simulink model "Appl_HeatAdj_CtrlModel"  (R2018b)
settings: configuration reference "CodeConfig_10_ms" (kept outside this file)
undefined symbols (not defined in the file): CAL_LEVEL3_TIMEOUT, CAL_SW_20min_TIMEOUT, D_1stLevel_36, D_2ndLevel_39, D_3rdLevel_45, D_3rdLevel_48, D_DRVHEAT_PID_D, D_DRVHEAT_PID_I, D_DRVHEAT_PID_P, D_HEAT_HEAT_DEF, D_SwsLevel_Temp, FALSE, TRUE
libraries: DareLib x111, simulink x1
(part 3 of 6)

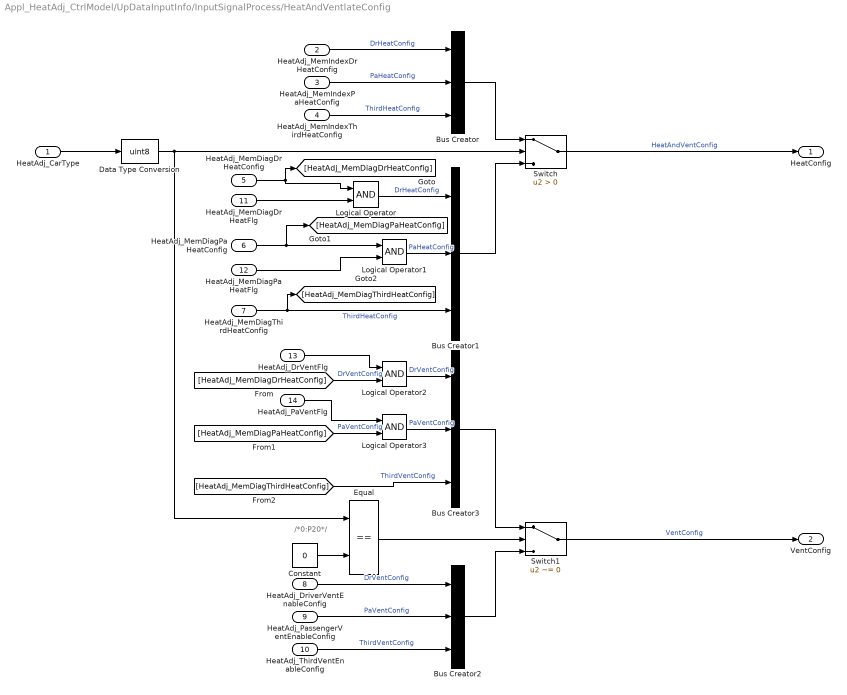
== system Appl_HeatAdj_CtrlModel/UpDataInputInfo/InputSignalProcess/HeatAndVentlateConfig ==
  note: /*0:P20*/
  HeatAdj_CarType : Inport
  HeatAdj_MemIndexDrHeatConfig : Inport  Port=2
  HeatAdj_MemIndexPaHeatConfig : Inport  Port=3
  HeatAdj_MemIndexThirdHeatConfig : Inport  Port=4
  HeatAdj_MemDiagDrHeatConfig : Inport  Port=5
  HeatAdj_MemDiagPaHeatConfig : Inport  Port=6
  HeatAdj_MemDiagThirdHeatConfig : Inport  Port=7
  HeatAdj_DriverVentEnableConfig : Inport  Port=8
  HeatAdj_PassengerVentEnableConfig : Inport  Port=9
  HeatAdj_ThirdVentEnableConfig : Inport  Port=10
  HeatAdj_MemDiagDrHeatFlg : Inport  Port=11
  HeatAdj_MemDiagPaHeatFlg : Inport  Port=12
  HeatAdj_DrVentFlg : Inport  Port=13
  HeatAdj_PaVentFlg : Inport  Port=14
  Bus Creator{,1..3} (4 alike) : BusCreator  Inputs=3
  Constant : Constant  Value=0  OutDataTypeStr=uint8
  Data Type Conversion : DataTypeConversion  OutDataTypeStr=uint8
  Equal : RelationalOperator  Operator===  OutDataTypeStr=boolean  RndMeth=Simplest
  Logical Operator{,1..3} (4 alike) : Logic  AllPortsSameDT=off  OutDataTypeStr=boolean
  Switch : Switch  Criteria=u2 > Threshold  OutDataTypeStr=uint8
  Switch1 : Switch  Criteria=u2 ~= 0
  HeatConfig : Outport
  VentConfig : Outport  Port=2
  wires:
  HeatAdj_CarType/1 -> Data Type Conversion/1
  HeatAdj_MemIndexDrHeatConfig/1 -> Bus Creator/1  "DrHeatConfig"
  HeatAdj_MemIndexPaHeatConfig/1 -> Bus Creator/2  "PaHeatConfig"
  HeatAdj_MemIndexThirdHeatConfig/1 -> Bus Creator/3  "ThirdHeatConfig"
  Bus Creator/1 -> Switch/1
  Bus Creator1/1 -> Switch/3
  HeatAdj_MemDiagDrHeatConfig/1 -> Logical Operator/1, [HeatAdj_MemDiagDrHeatConfig]
  HeatAdj_MemDiagPaHeatConfig/1 -> Logical Operator1/1, [HeatAdj_MemDiagPaHeatConfig]
  HeatAdj_MemDiagThirdHeatConfig/1 -> [HeatAdj_MemDiagThirdHeatConfig], Bus Creator1/3  "ThirdHeatConfig"
  Constant/1 -> Equal/2
  Equal/1 -> Switch1/2
  HeatAdj_DriverVentEnableConfig/1 -> Bus Creator2/1  "DrVentConfig"
  HeatAdj_PassengerVentEnableConfig/1 -> Bus Creator2/2  "PaVentConfig"
  HeatAdj_ThirdVentEnableConfig/1 -> Bus Creator2/3  "ThirdVentConfig"
  Bus Creator2/1 -> Switch1/3
  Switch/1 -> HeatConfig/1  "HeatAndVentConfig"
  Data Type Conversion/1 -> Switch/2, Equal/1
  Switch1/1 -> VentConfig/1  "VentConfig"
  [HeatAdj_MemDiagThirdHeatConfig] -> Bus Creator3/3  "ThirdVentConfig"
  [HeatAdj_MemDiagPaHeatConfig] -> Logical Operator3/2  "PaVentConfig"
  [HeatAdj_MemDiagDrHeatConfig] -> Logical Operator2/2  "DrVentConfig"
  Bus Creator3/1 -> Switch1/1
  HeatAdj_MemDiagDrHeatFlg/1 -> Logical Operator/2
  Logical Operator/1 -> Bus Creator1/1  "DrHeatConfig"
  HeatAdj_MemDiagPaHeatFlg/1 -> Logical Operator1/2
  Logical Operator1/1 -> Bus Creator1/2  "PaHeatConfig"
  HeatAdj_DrVentFlg/1 -> Logical Operator2/1
  Logical Operator2/1 -> Bus Creator3/1  "DrVentConfig"
  Logical Operator3/1 -> Bus Creator3/2  "PaVentConfig"
  HeatAdj_PaVentFlg/1 -> Logical Operator3/1

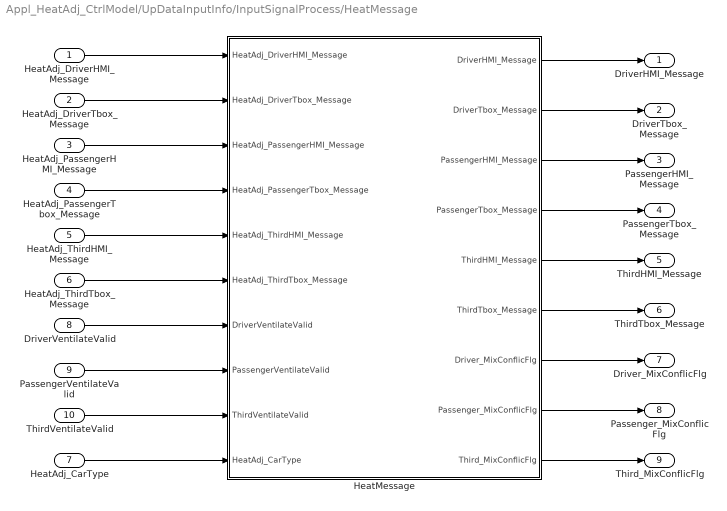
== system Appl_HeatAdj_CtrlModel/UpDataInputInfo/InputSignalProcess/HeatMessage ==
  HeatAdj_DriverHMI_Message : Inport
  HeatAdj_DriverTbox_Message : Inport  Port=2
  HeatAdj_PassengerHMI_Message : Inport  Port=3
  HeatAdj_PassengerTbox_Message : Inport  Port=4
  HeatAdj_ThirdHMI_Message : Inport  Port=5
  HeatAdj_ThirdTbox_Message : Inport  Port=6
  HeatAdj_CarType : Inport  Port=7
  DriverVentilateValid : Inport  Port=8
  PassengerVentilateValid : Inport  Port=9
  ThirdVentilateValid : Inport  Port=10
  HeatMessage : Stateflow chart  TreatAsAtomicUnit=on
  DriverHMI_Message : Outport
  DriverTbox_Message : Outport  Port=2
  PassengerHMI_Message : Outport  Port=3
  PassengerTbox_Message : Outport  Port=4
  ThirdHMI_Message : Outport  Port=5
  ThirdTbox_Message : Outport  Port=6
  Driver_MixConflicFlg : Outport  Port=7
  Passenger_MixConflicFlg : Outport  Port=8
  Third_MixConflicFlg : Outport  Port=9
  wires:
  HeatMessage/4(PassengerTbox_Message) -> PassengerTbox_Message/1
  HeatMessage/5(ThirdHMI_Message) -> ThirdHMI_Message/1
  HeatMessage/6(ThirdTbox_Message) -> ThirdTbox_Message/1
  ThirdVentilateValid/1 -> HeatMessage/9(ThirdVentilateValid)
  HeatAdj_DriverTbox_Message/1 -> HeatMessage/2(HeatAdj_DriverTbox_Message)
  HeatAdj_DriverHMI_Message/1 -> HeatMessage/1(HeatAdj_DriverHMI_Message)
  HeatAdj_PassengerHMI_Message/1 -> HeatMessage/3(HeatAdj_PassengerHMI_Message)
  HeatAdj_PassengerTbox_Message/1 -> HeatMessage/4(HeatAdj_PassengerTbox_Message)
  HeatAdj_ThirdHMI_Message/1 -> HeatMessage/5(HeatAdj_ThirdHMI_Message)
  PassengerVentilateValid/1 -> HeatMessage/8(PassengerVentilateValid)
  HeatAdj_ThirdTbox_Message/1 -> HeatMessage/6(HeatAdj_ThirdTbox_Message)
  DriverVentilateValid/1 -> HeatMessage/7(DriverVentilateValid)
  HeatMessage/1(DriverHMI_Message) -> DriverHMI_Message/1
  HeatMessage/2(DriverTbox_Message) -> DriverTbox_Message/1
  HeatMessage/3(PassengerHMI_Message) -> PassengerHMI_Message/1
  HeatAdj_CarType/1 -> HeatMessage/10(HeatAdj_CarType)
  HeatMessage/7(Driver_MixConflicFlg) -> Driver_MixConflicFlg/1
  HeatMessage/8(Passenger_MixConflicFlg) -> Passenger_MixConflicFlg/1
  HeatMessage/9(Third_MixConflicFlg) -> Third_MixConflicFlg/1

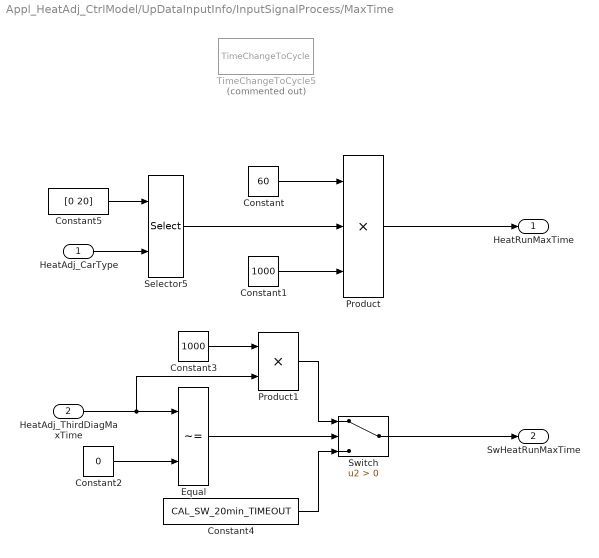
== system Appl_HeatAdj_CtrlModel/UpDataInputInfo/InputSignalProcess/MaxTime ==
  HeatAdj_CarType : Inport
  HeatAdj_ThirdDiagMaxTime : Inport  Port=2
  Constant : Constant  Value=60  OutDataTypeStr=uint32
  Constant1 : Constant  Value=1000  OutDataTypeStr=uint32
  Constant2 : Constant  Value=0  OutDataTypeStr=uint32
  Constant3 : Constant  Value=1000  OutDataTypeStr=uint32
  Constant4 : Constant  Value=CAL_SW_20min_TIMEOUT  OutDataTypeStr=uint32
  Constant5 : Constant  Value=[0 20]  OutDataTypeStr=uint32
  Equal : RelationalOperator  Operator=~=  OutDataTypeStr=boolean  RndMeth=Simplest
  Product : Product  Inputs=3  OutDataTypeStr=uint32
  Product1 : Product  OutDataTypeStr=uint32
  Selector5 : Selector  IndexMode=Zero-based  InputPortWidth=2  IndexOptions=Index vector (port)  Indices=[1 3]  OutputSizes=1
  Switch : Switch  Criteria=u2 > Threshold
  TimeChangeToCycle5 : DareLib/Dare/TimeChangeToCycle  Description=时间转成执行周期  Commented=on  Sec=60  Msec=1000  Cycle=CAL_HeatAdjCycle_10ms
      settings: AttributesFormatString=%<Description>  SourceProductName=Dare Library
  HeatRunMaxTime : Outport
  SwHeatRunMaxTime : Outport  Port=2
  wires:
  HeatAdj_CarType/1 -> Selector5/2
  Constant5/1 -> Selector5/1
  Selector5/1 -> Product/2
  Constant/1 -> Product/1
  Constant1/1 -> Product/3
  Product/1 -> HeatRunMaxTime/1
  HeatAdj_ThirdDiagMaxTime/1 -> Product1/2, Equal/1
  Constant2/1 -> Equal/2
  Equal/1 -> Switch/2
  Product1/1 -> Switch/1
  Constant3/1 -> Product1/1
  Constant4/1 -> Switch/3
  Switch/1 -> SwHeatRunMaxTime/1

== system Appl_HeatAdj_CtrlModel/UpDataInputInfo/InputSignalProcess/RemoteMode ==
  HeatAdj_RemoteEnableConfig : Inport
  HeatAdj_TboxRemoteSts : Inport  Port=2
  HeatAdj_RemoteMsgLostFlag : Inport  Port=3
  RemoteMode : Stateflow chart  TreatAsAtomicUnit=on
  RemoteModeFlag : Outport
  wires:
  HeatAdj_TboxRemoteSts/1 -> RemoteMode/2(HeatAdj_TboxRemoteSts)
  HeatAdj_RemoteEnableConfig/1 -> RemoteMode/1(HeatAdj_RemoteEnableConfig)
  HeatAdj_RemoteMsgLostFlag/1 -> RemoteMode/3(HeatAdj_RemoteMsgLostFlag)
  RemoteMode/1(RemoteModeFlag) -> RemoteModeFlag/1

== system Appl_HeatAdj_CtrlModel/UpDataInputInfo/InputSignalProcess/VehRunSta ==
  HeatAdj_PlatformVehicleEnableConfig : Inport
  HeatAdj_P20_PHEV_EngineCfg : Inport  Port=2
  HeatAdj_VCU_VehRunSta : Inport  Port=3
  HeatAdj_CarType : Inport  Port=4
  VehicleRunStatus : Stateflow chart  TreatAsAtomicUnit=on
  "VehicleRunFlag " : Outport
  wires:
  HeatAdj_VCU_VehRunSta/1 -> VehicleRunStatus/3(HeatAdj_VCU_VehRunSta)
  HeatAdj_PlatformVehicleEnableConfig/1 -> VehicleRunStatus/1(HeatAdj_PlatformVehicleEnableConfig)
  HeatAdj_P20_PHEV_EngineCfg/1 -> VehicleRunStatus/2(HeatAdj_P20_PHEV_EngineCfg)
  VehicleRunStatus/1(VehicleRunFlag) -> "VehicleRunFlag "/1
  HeatAdj_CarType/1 -> VehicleRunStatus/4(HeatAdj_CarType)

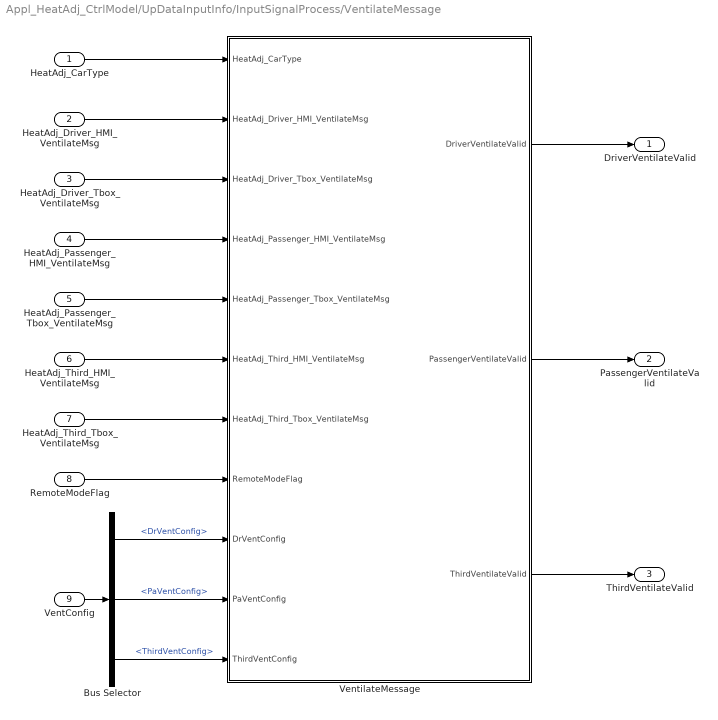
== system Appl_HeatAdj_CtrlModel/UpDataInputInfo/InputSignalProcess/VentilateMessage ==
  HeatAdj_CarType : Inport
  HeatAdj_Driver_HMI_VentilateMsg : Inport  Port=2
  HeatAdj_Driver_Tbox_VentilateMsg : Inport  Port=3
  HeatAdj_Passenger_HMI_VentilateMsg : Inport  Port=4
  HeatAdj_Passenger_Tbox_VentilateMsg : Inport  Port=5
  HeatAdj_Third_HMI_VentilateMsg : Inport  Port=6
  HeatAdj_Third_Tbox_VentilateMsg : Inport  Port=7
  RemoteModeFlag : Inport  Port=8
  VentConfig : Inport  Port=9
  Bus Selector : BusSelector  OutputSignals=DrVentConfig,PaVentConfig,ThirdVentConfig
  VentilateMessage : Stateflow chart  TreatAsAtomicUnit=on
  DriverVentilateValid : Outport
  PassengerVentilateValid : Outport  Port=2
  ThirdVentilateValid : Outport  Port=3
  wires:
  HeatAdj_Driver_HMI_VentilateMsg/1 -> VentilateMessage/2(HeatAdj_Driver_HMI_VentilateMsg)
  HeatAdj_CarType/1 -> VentilateMessage/1(HeatAdj_CarType)
  HeatAdj_Driver_Tbox_VentilateMsg/1 -> VentilateMessage/3(HeatAdj_Driver_Tbox_VentilateMsg)
  HeatAdj_Passenger_HMI_VentilateMsg/1 -> VentilateMessage/4(HeatAdj_Passenger_HMI_VentilateMsg)
  HeatAdj_Passenger_Tbox_VentilateMsg/1 -> VentilateMessage/5(HeatAdj_Passenger_Tbox_VentilateMsg)
  RemoteModeFlag/1 -> VentilateMessage/8(RemoteModeFlag)
  HeatAdj_Third_HMI_VentilateMsg/1 -> VentilateMessage/6(HeatAdj_Third_HMI_VentilateMsg)
  HeatAdj_Third_Tbox_VentilateMsg/1 -> VentilateMessage/7(HeatAdj_Third_Tbox_VentilateMsg)
  VentilateMessage/1(DriverVentilateValid) -> DriverVentilateValid/1
  VentilateMessage/2(PassengerVentilateValid) -> PassengerVentilateValid/1
  VentilateMessage/3(ThirdVentilateValid) -> ThirdVentilateValid/1
  VentConfig/1 -> Bus Selector/1
  Bus Selector/1 -> VentilateMessage/9(DrVentConfig)  "<DrVentConfig>"
  Bus Selector/2 -> VentilateMessage/10(PaVentConfig)  "<PaVentConfig>"
  Bus Selector/3 -> VentilateMessage/11(ThirdVentConfig)  "<ThirdVentConfig>"

== system Appl_HeatAdj_CtrlModel/LogicCtrl/LocalAdjustCtrl/LimitDeal/TimeoutFunction/Timeout/D_HAL_GET_CUR_MS_TS ==
  f : TriggerPort  TriggerType=function-call  VariantControl=(inherit)
      settings: CopyFcn=Stateflow.SLINSF.SimulinkMan.removeBlockPreDeleteFcn  PreDeleteFcn=Stateflow.SLINSF.SimulinkMan.unsafePredeleteFcn
  DrAdj_LenAdjSize : DareLib/Dare/getAPI_type  g_funcname=D_HAL_GET_CUR_MS_TS  g_param=""  g_type=uint32  g_size=-1
      settings: SourceProductName=Dare Library
  Ts : Outport
  wires:
  DrAdj_LenAdjSize/1 -> Ts/1  "D_HAL_GET_CUR_MS_TS"

== system Appl_HeatAdj_CtrlModel/LogicCtrl/LocalAdjustCtrl/LimitDeal/TimeoutFunction/Timeout/TimeDiffTs ==
  lastTs : Inport
  Ts : Inport  Port=2
  f : TriggerPort  TriggerType=function-call  VariantControl=(inherit)
      settings: CopyFcn=Stateflow.SLINSF.SimulinkMan.removeBlockPreDeleteFcn  PreDeleteFcn=Stateflow.SLINSF.SimulinkMan.unsafePredeleteFcn
  Chart : Stateflow chart  TreatAsAtomicUnit=on
  OutTs : Outport
  wires:
  lastTs/1 -> Chart/1(lastTs)
  Ts/1 -> Chart/2(Ts)
  Chart/1(OutTs) -> OutTs/1

== system Appl_HeatAdj_CtrlModel/LogicCtrl/LocalAdjustCtrl/LimitDeal/TimeoutFunction1/Timeout/D_HAL_GET_CUR_MS_TS ==
  f : TriggerPort  TriggerType=function-call  VariantControl=(inherit)
      settings: CopyFcn=Stateflow.SLINSF.SimulinkMan.removeBlockPreDeleteFcn  PreDeleteFcn=Stateflow.SLINSF.SimulinkMan.unsafePredeleteFcn
  DrAdj_LenAdjSize : DareLib/Dare/getAPI_type  g_funcname=D_HAL_GET_CUR_MS_TS  g_param=""  g_type=uint32  g_size=-1
      settings: SourceProductName=Dare Library
  Ts : Outport
  wires:
  DrAdj_LenAdjSize/1 -> Ts/1  "D_HAL_GET_CUR_MS_TS"

== system Appl_HeatAdj_CtrlModel/LogicCtrl/LocalAdjustCtrl/LimitDeal/TimeoutFunction1/Timeout/TimeDiffTs ==
  lastTs : Inport
  Ts : Inport  Port=2
  f : TriggerPort  TriggerType=function-call  VariantControl=(inherit)
      settings: CopyFcn=Stateflow.SLINSF.SimulinkMan.removeBlockPreDeleteFcn  PreDeleteFcn=Stateflow.SLINSF.SimulinkMan.unsafePredeleteFcn
  Chart : Stateflow chart  TreatAsAtomicUnit=on
  OutTs : Outport
  wires:
  lastTs/1 -> Chart/1(lastTs)
  Ts/1 -> Chart/2(Ts)
  Chart/1(OutTs) -> OutTs/1

== system Appl_HeatAdj_CtrlModel/LogicCtrl/LocalAdjustCtrl/OutputDeal/HeatOutFunction/HeatOut/PidGetPwm ==
  CurrentTemp : Inport
  SetTemp : Inport  Port=2
  f : TriggerPort  TriggerType=function-call  VariantControl=(inherit)
      settings: CopyFcn=Stateflow.SLINSF.SimulinkMan.removeBlockPreDeleteFcn  PreDeleteFcn=Stateflow.SLINSF.SimulinkMan.unsafePredeleteFcn
  "Pid " : Stateflow chart  TreatAsAtomicUnit=on
  PwmCnt : Outport
  wires:
  CurrentTemp/1 -> "Pid "/1(CurrentTemp)
  SetTemp/1 -> "Pid "/2(SetTemp)
  "Pid "/1(PwmCnt) -> PwmCnt/1

== system Appl_HeatAdj_CtrlModel/LogicCtrl/LocalAdjustCtrl/OutputDeal/HeatOutFunction1/HeatOut/PidGetPwm ==
  CurrentTemp : Inport
  SetTemp : Inport  Port=2
  f : TriggerPort  TriggerType=function-call  VariantControl=(inherit)
      settings: CopyFcn=Stateflow.SLINSF.SimulinkMan.removeBlockPreDeleteFcn  PreDeleteFcn=Stateflow.SLINSF.SimulinkMan.unsafePredeleteFcn
  "Pid " : Stateflow chart  TreatAsAtomicUnit=on
  PwmCnt : Outport
  wires:
  CurrentTemp/1 -> "Pid "/1(CurrentTemp)
  SetTemp/1 -> "Pid "/2(SetTemp)
  "Pid "/1(PwmCnt) -> PwmCnt/1

== system Appl_HeatAdj_CtrlModel/LogicCtrl/LocalAdjustCtrl/OutputDeal/HeatOutFunction2/HeatOut/D_HAL_GET_CUR_MS_TS ==
  f : TriggerPort  TriggerType=function-call  VariantControl=(inherit)
      settings: CopyFcn=Stateflow.SLINSF.SimulinkMan.removeBlockPreDeleteFcn  PreDeleteFcn=Stateflow.SLINSF.SimulinkMan.unsafePredeleteFcn
  DrAdj_LenAdjSize : DareLib/Dare/getAPI_type  g_funcname=D_HAL_GET_CUR_MS_TS  g_param=""  g_type=uint32  g_size=-1
      settings: SourceProductName=Dare Library
  Ts : Outport
  wires:
  DrAdj_LenAdjSize/1 -> Ts/1  "D_HAL_GET_CUR_MS_TS"

== system Appl_HeatAdj_CtrlModel/LogicCtrl/LocalAdjustCtrl/OutputDeal/HeatOutFunction2/HeatOut/PidGetPwm ==
  CurrentTemp : Inport
  SetTemp : Inport  Port=2
  f : TriggerPort  TriggerType=function-call  VariantControl=(inherit)
      settings: CopyFcn=Stateflow.SLINSF.SimulinkMan.removeBlockPreDeleteFcn  PreDeleteFcn=Stateflow.SLINSF.SimulinkMan.unsafePredeleteFcn
  "Pid " : Stateflow chart  TreatAsAtomicUnit=on
  PwmCnt : Outport
  wires:
  CurrentTemp/1 -> "Pid "/1(CurrentTemp)
  SetTemp/1 -> "Pid "/2(SetTemp)
  "Pid "/1(PwmCnt) -> PwmCnt/1

== system Appl_HeatAdj_CtrlModel/LogicCtrl/LocalAdjustCtrl/OutputDeal/HeatOutFunction2/HeatOut/TimeDiffTs ==
  lastTs : Inport
  Ts : Inport  Port=2
  f : TriggerPort  TriggerType=function-call  VariantControl=(inherit)
      settings: CopyFcn=Stateflow.SLINSF.SimulinkMan.removeBlockPreDeleteFcn  PreDeleteFcn=Stateflow.SLINSF.SimulinkMan.unsafePredeleteFcn
  Chart : Stateflow chart  TreatAsAtomicUnit=on
  OutTs : Outport
  wires:
  lastTs/1 -> Chart/1(lastTs)
  Ts/1 -> Chart/2(Ts)
  Chart/1(OutTs) -> OutTs/1

== system Appl_HeatAdj_CtrlModel/LogicCtrl/LocalAdjustCtrl/OutputDeal/TempFunction/TempFunction/D_HAL_GET_CUR_MS_TS ==
  f : TriggerPort  TriggerType=function-call  VariantControl=(inherit)
      settings: CopyFcn=Stateflow.SLINSF.SimulinkMan.removeBlockPreDeleteFcn  PreDeleteFcn=Stateflow.SLINSF.SimulinkMan.unsafePredeleteFcn
  DrAdj_LenAdjSize : DareLib/Dare/getAPI_type  g_funcname=D_HAL_GET_CUR_MS_TS  g_param=""  g_type=uint32  g_size=-1
      settings: SourceProductName=Dare Library
  Ts : Outport
  wires:
  DrAdj_LenAdjSize/1 -> Ts/1  "D_HAL_GET_CUR_MS_TS"

== system Appl_HeatAdj_CtrlModel/LogicCtrl/LocalAdjustCtrl/OutputDeal/TempFunction/TempFunction/TimeDiffTs ==
  lastTs : Inport
  Ts : Inport  Port=2
  f : TriggerPort  TriggerType=function-call  VariantControl=(inherit)
      settings: CopyFcn=Stateflow.SLINSF.SimulinkMan.removeBlockPreDeleteFcn  PreDeleteFcn=Stateflow.SLINSF.SimulinkMan.unsafePredeleteFcn
  Chart : Stateflow chart  TreatAsAtomicUnit=on
  OutTs : Outport
  wires:
  lastTs/1 -> Chart/1(lastTs)
  Ts/1 -> Chart/2(Ts)
  Chart/1(OutTs) -> OutTs/1

== system Appl_HeatAdj_CtrlModel/LogicCtrl/LocalAdjustCtrl/OutputDeal/TempFunction1/TempFunction/D_HAL_GET_CUR_MS_TS ==
  f : TriggerPort  TriggerType=function-call  VariantControl=(inherit)
      settings: CopyFcn=Stateflow.SLINSF.SimulinkMan.removeBlockPreDeleteFcn  PreDeleteFcn=Stateflow.SLINSF.SimulinkMan.unsafePredeleteFcn
  DrAdj_LenAdjSize : DareLib/Dare/getAPI_type  g_funcname=D_HAL_GET_CUR_MS_TS  g_param=""  g_type=uint32  g_size=-1
      settings: SourceProductName=Dare Library
  Ts : Outport
  wires:
  DrAdj_LenAdjSize/1 -> Ts/1  "D_HAL_GET_CUR_MS_TS"

== system Appl_HeatAdj_CtrlModel/LogicCtrl/LocalAdjustCtrl/OutputDeal/TempFunction1/TempFunction/TimeDiffTs ==
  lastTs : Inport
  Ts : Inport  Port=2
  f : TriggerPort  TriggerType=function-call  VariantControl=(inherit)
      settings: CopyFcn=Stateflow.SLINSF.SimulinkMan.removeBlockPreDeleteFcn  PreDeleteFcn=Stateflow.SLINSF.SimulinkMan.unsafePredeleteFcn
  Chart : Stateflow chart  TreatAsAtomicUnit=on
  OutTs : Outport
  wires:
  lastTs/1 -> Chart/1(lastTs)
  Ts/1 -> Chart/2(Ts)
  Chart/1(OutTs) -> OutTs/1

== system Appl_HeatAdj_CtrlModel/LogicCtrl/LocalAdjustCtrl/OutputDeal/TempFunction2/TempFunction/D_HAL_GET_CUR_MS_TS ==
  f : TriggerPort  TriggerType=function-call  VariantControl=(inherit)
      settings: CopyFcn=Stateflow.SLINSF.SimulinkMan.removeBlockPreDeleteFcn  PreDeleteFcn=Stateflow.SLINSF.SimulinkMan.unsafePredeleteFcn
  DrAdj_LenAdjSize : DareLib/Dare/getAPI_type  g_funcname=D_HAL_GET_CUR_MS_TS  g_param=""  g_type=uint32  g_size=-1
      settings: SourceProductName=Dare Library
  Ts : Outport
  wires:
  DrAdj_LenAdjSize/1 -> Ts/1  "D_HAL_GET_CUR_MS_TS"

== system Appl_HeatAdj_CtrlModel/LogicCtrl/LocalAdjustCtrl/OutputDeal/TempFunction2/TempFunction/TimeDiffTs ==
  lastTs : Inport
  Ts : Inport  Port=2
  f : TriggerPort  TriggerType=function-call  VariantControl=(inherit)
      settings: CopyFcn=Stateflow.SLINSF.SimulinkMan.removeBlockPreDeleteFcn  PreDeleteFcn=Stateflow.SLINSF.SimulinkMan.unsafePredeleteFcn
  Chart : Stateflow chart  TreatAsAtomicUnit=on
  OutTs : Outport
  wires:
  lastTs/1 -> Chart/1(lastTs)
  Ts/1 -> Chart/2(Ts)
  Chart/1(OutTs) -> OutTs/1

== system Appl_HeatAdj_CtrlModel/UpDataInputInfo/InputSignalProcess/EorrorProcess/EorrorProcess/ErrorFunction ==
  FirstFaultSts : Inport
  SecondFaultSts : Inport  Port=2
  f : TriggerPort  TriggerType=function-call  VariantControl=(inherit)
      settings: CopyFcn=Stateflow.SLINSF.SimulinkMan.removeBlockPreDeleteFcn  PreDeleteFcn=Stateflow.SLINSF.SimulinkMan.unsafePredeleteFcn
  OppositeMessageDeal : Stateflow chart  TreatAsAtomicUnit=on
  "HeatError " : Outport
  wires:
  OppositeMessageDeal/1(HeatErr) -> "HeatError "/1
  FirstFaultSts/1 -> OppositeMessageDeal/1(FirstFaultSts)
  SecondFaultSts/1 -> OppositeMessageDeal/2(SecondFaultSts)

== system Appl_HeatAdj_CtrlModel/UpDataInputInfo/InputSignalProcess/EorrorProcess/EorrorProcess/ErrorFunction1 ==
  FirstFaultSts : Inport
  SecondFaultSts : Inport  Port=2
  f : TriggerPort  TriggerType=function-call  VariantControl=(inherit)
      settings: CopyFcn=Stateflow.SLINSF.SimulinkMan.removeBlockPreDeleteFcn  PreDeleteFcn=Stateflow.SLINSF.SimulinkMan.unsafePredeleteFcn
  OppositeMessageDeal : Stateflow chart  TreatAsAtomicUnit=on
  "HeatError " : Outport
  wires:
  OppositeMessageDeal/1(HeatErr) -> "HeatError "/1
  FirstFaultSts/1 -> OppositeMessageDeal/1(FirstFaultSts)
  SecondFaultSts/1 -> OppositeMessageDeal/2(SecondFaultSts)

== system Appl_HeatAdj_CtrlModel/UpDataInputInfo/InputSignalProcess/EorrorProcess/EorrorProcess/ErrorFunction2 ==
  FirstFaultSts : Inport
  SecondFaultSts : Inport  Port=2
  f : TriggerPort  TriggerType=function-call  VariantControl=(inherit)
      settings: CopyFcn=Stateflow.SLINSF.SimulinkMan.removeBlockPreDeleteFcn  PreDeleteFcn=Stateflow.SLINSF.SimulinkMan.unsafePredeleteFcn
  OppositeMessageDeal : Stateflow chart  TreatAsAtomicUnit=on
  "HeatError " : Outport
  wires:
  OppositeMessageDeal/1(HeatErr) -> "HeatError "/1
  FirstFaultSts/1 -> OppositeMessageDeal/1(FirstFaultSts)
  SecondFaultSts/1 -> OppositeMessageDeal/2(SecondFaultSts)

== system Appl_HeatAdj_CtrlModel/UpDataInputInfo/InputSignalProcess/EorrorProcess/EorrorProcess/ErrorFunction3 ==
  FirstFaultSts : Inport
  SecondFaultSts : Inport  Port=2
  f : TriggerPort  TriggerType=function-call  VariantControl=(inherit)
      settings: CopyFcn=Stateflow.SLINSF.SimulinkMan.removeBlockPreDeleteFcn  PreDeleteFcn=Stateflow.SLINSF.SimulinkMan.unsafePredeleteFcn
  OppositeMessageDeal : Stateflow chart  TreatAsAtomicUnit=on
  "HeatError " : Outport
  wires:
  OppositeMessageDeal/1(HeatErr) -> "HeatError "/1
  FirstFaultSts/1 -> OppositeMessageDeal/1(FirstFaultSts)
  SecondFaultSts/1 -> OppositeMessageDeal/2(SecondFaultSts)

== system Appl_HeatAdj_CtrlModel/UpDataInputInfo/InputSignalProcess/EorrorProcess/EorrorProcess/ErrorFunction4 ==
  FirstFaultSts : Inport
  SecondFaultSts : Inport  Port=2
  f : TriggerPort  TriggerType=function-call  VariantControl=(inherit)
      settings: CopyFcn=Stateflow.SLINSF.SimulinkMan.removeBlockPreDeleteFcn  PreDeleteFcn=Stateflow.SLINSF.SimulinkMan.unsafePredeleteFcn
  OppositeMessageDeal : Stateflow chart  TreatAsAtomicUnit=on
  "HeatError " : Outport
  wires:
  OppositeMessageDeal/1(HeatErr) -> "HeatError "/1
  FirstFaultSts/1 -> OppositeMessageDeal/1(FirstFaultSts)
  SecondFaultSts/1 -> OppositeMessageDeal/2(SecondFaultSts)

== system Appl_HeatAdj_CtrlModel/UpDataInputInfo/InputSignalProcess/EorrorProcess/EorrorProcess/ErrorFunction5 ==
  FirstFaultSts : Inport
  SecondFaultSts : Inport  Port=2
  f : TriggerPort  TriggerType=function-call  VariantControl=(inherit)
      settings: CopyFcn=Stateflow.SLINSF.SimulinkMan.removeBlockPreDeleteFcn  PreDeleteFcn=Stateflow.SLINSF.SimulinkMan.unsafePredeleteFcn
  OppositeMessageDeal : Stateflow chart  TreatAsAtomicUnit=on
  "HeatError " : Outport
  wires:
  OppositeMessageDeal/1(HeatErr) -> "HeatError "/1
  FirstFaultSts/1 -> OppositeMessageDeal/1(FirstFaultSts)
  SecondFaultSts/1 -> OppositeMessageDeal/2(SecondFaultSts)

== system Appl_HeatAdj_CtrlModel/UpDataInputInfo/InputSignalProcess/HeatMessage/HeatMessage/MsgConflictFunction ==
  CarTypeCfg : Inport
  HMI_Message : Inport  Port=2  OutDataTypeStr=uint8
  Tbox_Message : Inport  Port=3  OutDataTypeStr=uint8
  VentValidFlag : Inport  Port=4
  f : TriggerPort  TriggerType=function-call  VariantControl=(inherit)
      settings: CopyFcn=Stateflow.SLINSF.SimulinkMan.removeBlockPreDeleteFcn  PreDeleteFcn=Stateflow.SLINSF.SimulinkMan.unsafePredeleteFcn
  Function : Stateflow chart  TreatAsAtomicUnit=on
  OutMsgHMI : Outport
  OutMsgTbox : Outport  Port=2
  MixConflictFlg : Outport  Port=3
  wires:
  Function/1(OutMsgHMI) -> OutMsgHMI/1
  VentValidFlag/1 -> Function/4(VentValidFlag)
  CarTypeCfg/1 -> Function/1(CarTypeCfg)
  HMI_Message/1 -> Function/2(HMI_Message)
  Tbox_Message/1 -> Function/3(Tbox_Message)
  Function/2(OutMsgTbox) -> OutMsgTbox/1
  Function/3(MixConflictFlg) -> MixConflictFlg/1

== system Appl_HeatAdj_CtrlModel/UpDataInputInfo/InputSignalProcess/HeatMessage/HeatMessage/MsgConflictFunction1 ==
  CarTypeCfg : Inport
  HMI_Message : Inport  Port=2  OutDataTypeStr=uint8
  Tbox_Message : Inport  Port=3  OutDataTypeStr=uint8
  VentValidFlag : Inport  Port=4
  f : TriggerPort  TriggerType=function-call  VariantControl=(inherit)
      settings: CopyFcn=Stateflow.SLINSF.SimulinkMan.removeBlockPreDeleteFcn  PreDeleteFcn=Stateflow.SLINSF.SimulinkMan.unsafePredeleteFcn
  Function : Stateflow chart  TreatAsAtomicUnit=on
  OutMsgHMI : Outport
  OutMsgTbox : Outport  Port=2
  MixConflictFlg : Outport  Port=3
  wires:
  Function/1(OutMsgHMI) -> OutMsgHMI/1
  VentValidFlag/1 -> Function/4(VentValidFlag)
  CarTypeCfg/1 -> Function/1(CarTypeCfg)
  HMI_Message/1 -> Function/2(HMI_Message)
  Tbox_Message/1 -> Function/3(Tbox_Message)
  Function/2(OutMsgTbox) -> OutMsgTbox/1
  Function/3(MixConflictFlg) -> MixConflictFlg/1

== system Appl_HeatAdj_CtrlModel/UpDataInputInfo/InputSignalProcess/HeatMessage/HeatMessage/MsgConflictFunction2 ==
  CarTypeCfg : Inport
  HMI_Message : Inport  Port=2  OutDataTypeStr=uint8
  Tbox_Message : Inport  Port=3  OutDataTypeStr=uint8
  VentValidFlag : Inport  Port=4
  f : TriggerPort  TriggerType=function-call  VariantControl=(inherit)
      settings: CopyFcn=Stateflow.SLINSF.SimulinkMan.removeBlockPreDeleteFcn  PreDeleteFcn=Stateflow.SLINSF.SimulinkMan.unsafePredeleteFcn
  Function : Stateflow chart  TreatAsAtomicUnit=on
  OutMsgHMI : Outport
  OutMsgTbox : Outport  Port=2
  MixConflictFlg : Outport  Port=3
  wires:
  Function/1(OutMsgHMI) -> OutMsgHMI/1
  VentValidFlag/1 -> Function/4(VentValidFlag)
  CarTypeCfg/1 -> Function/1(CarTypeCfg)
  HMI_Message/1 -> Function/2(HMI_Message)
  Tbox_Message/1 -> Function/3(Tbox_Message)
  Function/2(OutMsgTbox) -> OutMsgTbox/1
  Function/3(MixConflictFlg) -> MixConflictFlg/1

== system Appl_HeatAdj_CtrlModel/UpDataInputInfo/InputSignalProcess/VentilateMessage/VentilateMessage/OppositeMessageDeal ==
  CarTypeCfg : Inport
  RemoteModeFlag : Inport  Port=2
  HMI_Message : Inport  Port=3
  Tbox_Message : Inport  Port=4
  VentCfg : Inport  Port=5
  f : TriggerPort  TriggerType=function-call  VariantControl=(inherit)
      settings: CopyFcn=Stateflow.SLINSF.SimulinkMan.removeBlockPreDeleteFcn  PreDeleteFcn=Stateflow.SLINSF.SimulinkMan.unsafePredeleteFcn
  OppositeMessageDeal : Stateflow chart  TreatAsAtomicUnit=on
  "VenSts " : Outport
  wires:
  RemoteModeFlag/1 -> OppositeMessageDeal/2(RemoteModeFlag)
  HMI_Message/1 -> OppositeMessageDeal/3(HMI_Message)
  CarTypeCfg/1 -> OppositeMessageDeal/1(CarTypeCfg)
  Tbox_Message/1 -> OppositeMessageDeal/4(Tbox_Message)
  OppositeMessageDeal/1(VenSts) -> "VenSts "/1
  VentCfg/1 -> OppositeMessageDeal/5(VentCfg)

== system Appl_HeatAdj_CtrlModel/UpDataInputInfo/InputSignalProcess/VentilateMessage/VentilateMessage/OppositeMessageDeal1 ==
  CarTypeCfg : Inport
  RemoteModeFlag : Inport  Port=2
  HMI_Message : Inport  Port=3
  Tbox_Message : Inport  Port=4
  VentCfg : Inport  Port=5
  f : TriggerPort  TriggerType=function-call  VariantControl=(inherit)
      settings: CopyFcn=Stateflow.SLINSF.SimulinkMan.removeBlockPreDeleteFcn  PreDeleteFcn=Stateflow.SLINSF.SimulinkMan.unsafePredeleteFcn
  OppositeMessageDeal : Stateflow chart  TreatAsAtomicUnit=on
  "VenSts " : Outport
  wires:
  RemoteModeFlag/1 -> OppositeMessageDeal/2(RemoteModeFlag)
  HMI_Message/1 -> OppositeMessageDeal/3(HMI_Message)
  CarTypeCfg/1 -> OppositeMessageDeal/1(CarTypeCfg)
  Tbox_Message/1 -> OppositeMessageDeal/4(Tbox_Message)
  OppositeMessageDeal/1(VenSts) -> "VenSts "/1
  VentCfg/1 -> OppositeMessageDeal/5(VentCfg)

== system Appl_HeatAdj_CtrlModel/UpDataInputInfo/InputSignalProcess/VentilateMessage/VentilateMessage/OppositeMessageDeal2 ==
  CarTypeCfg : Inport
  RemoteModeFlag : Inport  Port=2
  HMI_Message : Inport  Port=3
  Tbox_Message : Inport  Port=4
  VentCfg : Inport  Port=5
  f : TriggerPort  TriggerType=function-call  VariantControl=(inherit)
      settings: CopyFcn=Stateflow.SLINSF.SimulinkMan.removeBlockPreDeleteFcn  PreDeleteFcn=Stateflow.SLINSF.SimulinkMan.unsafePredeleteFcn
  OppositeMessageDeal : Stateflow chart  TreatAsAtomicUnit=on
  "VenSts " : Outport
  wires:
  RemoteModeFlag/1 -> OppositeMessageDeal/2(RemoteModeFlag)
  HMI_Message/1 -> OppositeMessageDeal/3(HMI_Message)
  CarTypeCfg/1 -> OppositeMessageDeal/1(CarTypeCfg)
  Tbox_Message/1 -> OppositeMessageDeal/4(Tbox_Message)
  OppositeMessageDeal/1(VenSts) -> "VenSts "/1
  VentCfg/1 -> OppositeMessageDeal/5(VentCfg)

== stateflow chart Appl_HeatAdj_CtrlModel/LogicCtrl/LocalAdjustCtrl/HeatLevelDeal/LevelAquireFunction1/LevelAquireFunction ==
  state LevelAquire
    (default) -> (junction 103)
    LevelAquire -> (junction 103)
    (junction 103) -> (junction 105) [order 1] : /*加热功能禁能
        | || 通用前置条件不满足)*/
        | [enHeatStopReason.EN_HEAT_STOP_R_NONE != DisableSts ...
        | || FALSE == EnableCfg ...
        | || TRUE != ComPCFlag]
    (junction 103) -> (junction 102) [order 2] : {StopFlag = FALSE;}
    (junction 105) -> (junction 104) : {Level = enHeatLvlSts.EN_HEAT_LVL_OFF;
        | StopFlag = TRUE;}
    (junction 104) -> (junction 102)
    (junction 102) -> (junction 111)
    (junction 111) -> (junction 21) [order 1] : [FALSE == StopFlag]
    (junction 21) -> (junction 23) [order 1] : [enProjectType.EN_PROJECT_P20 == CarTypeCfg]
    (junction 111) -> (junction 114) [order 2] : {Level = enHeatLvlSts.EN_HEAT_LVL_OFF;}
    (junction 21) -> (junction 48) [order 2]
    (junction 23) -> (junction 85)
    (junction 85) -> (junction 87) [order 1] : /* open 信号 且为HMI控制*/
        | [5 == CAN_Message && Type == FALSE]
    (junction 85) -> (junction 25) [order 2]
    (junction 87) -> (junction 89) : {Level = CanLvl + 1;}
    (junction 25) -> (junction 27) [order 1] : [4 == CAN_Message]
    (junction 25) -> (junction 29) [order 2] : {TempMsg = CAN_Message + 1;}
    (junction 27) -> (junction 57) : {Level = enHeatLvlSts.EN_HEAT_LVL_OFF;}
    (junction 48) -> (junction 50) [order 1] : [1 != CAN_Message]
    (junction 48) -> (junction 55) [order 2] : {Level = enHeatLvlSts.EN_HEAT_LVL_OFF;}
    (junction 50) -> (junction 52) : {TempMsg = CAN_Message;}
    (junction 52) -> (junction 29)
    (junction 29) -> (junction 32) [order 1] : [1 < TempMsg && 5 > TempMsg]
    (junction 29) -> (junction 36) [order 2] : {Level = 0xFF;}
    (junction 32) -> (junction 34)
    (junction 34) -> (junction 38) [order 1] : [2 == TempMsg]
    (junction 34) -> (junction 40) [order 2]
    (junction 38) -> (junction 59) : {Level = enHeatLvlSts.EN_HEAT_LVL_1;}
    (junction 40) -> (junction 42) [order 1] : [3 == TempMsg]
    (junction 40) -> (junction 46) [order 2] : {Level = enHeatLvlSts.EN_HEAT_LVL_3;}
    (junction 42) -> (junction 44) : {Level = enHeatLvlSts.EN_HEAT_LVL_2;}
    (junction 55) -> (junction 114)
    (junction 36) -> (junction 55)
    (junction 46) -> (junction 36)
    (junction 44) -> (junction 46)
    (junction 59) -> (junction 44)
    (junction 57) -> (junction 59)
    (junction 89) -> (junction 57)
    (junction 114) -> (junction 75)
  data: EnableCfg input uint8; CarTypeCfg input Enum: enProjectType; CAN_Message input uint8; DisableSts input Enum: enHeatStopReason; Level output uint8; TempMsg local uint8; TRUE parameter; FALSE parameter; ComPCFlag input; CanLvl input uint8; Type input; CurLvl input; StopFlag local boolean

== stateflow chart Appl_HeatAdj_CtrlModel/LogicCtrl/LocalAdjustCtrl/LimitDeal ==
  state OutValid = MixConflic(MixFlg,Valid) [function]
  state MixConflic1 [parallel]
    en,du:
    [LocalDriverVentilateValid] = MixConflic(Driver_MixConflicFlg, DriverVentilateValid);
    [LocalPassengerVentilateValid] = MixConflic(Passenger_MixConflicFlg, PassengerVentilateValid);
    [LocalThirdVentilateValid] = MixConflic(Third_MixConflicFlg, ThirdVentilateValid);
    settings: executionOrder=1
  state [Level,StopReason,CANStopReason] = LevelLimitFunction(OriginalLevel,Error,OppositeCmd,CarType,Heat_CanMessageLostFlag,Heat_RecoverDefaultFlag) [function]
  state ForbidLimitDeal [parallel]
    en,du:
    [ComDrHeatLevel,ComDrStopReason,ComCANDrStopReason] = LevelLimitFunction(OriginalDrHeatLevel,DriverHeatError, LocalDriverVentilateValid,HeatAdj_CarType,HeatAdj_HeatMsgLostFlag,HeatAdj_RecoverDefaultFlag);
    [ComPaHeatLevel,ComPaStopReason,ComCANPaStopReason] = LevelLimitFunction1(OriginalPaHeatLevel,PassengerHeatError, LocalPassengerVentilateValid,HeatAdj_CarType,HeatAdj_HeatMsgLostFlag,HeatAdj_RecoverDefaultFlag);
    [Com3rdHeatLevel,Com3rdStopReason,ComCAN3rdStopReason] = LevelLimitFunction2(Original3rdHeatLevel,ThirdHeatError, LocalThirdVentilateValid,HeatAdj_CarType,HeatAdj_HeatMsgLostFlag,HeatAdj_RecoverDefaultFlag);
    settings: executionOrder=2
  state [Level,StopReason,CANStopReason] = LevelLimitFunction1(OriginalLevel,Error,OppositeCmd,CarType,Heat_CanMessageLostFlag,Heat_RecoverDefaultFlag) [function]
  state [Level,StopReason,CANStopReason] = LevelLimitFunction2(OriginalLevel,Error,OppositeCmd,CarType,Heat_CanMessageLostFlag,Heat_RecoverDefaultFlag) [function]
  state [Level,TimeoutFlag] = TimeoutFunction(TimeoutPrm,MaxTime,InLevel) [function]
  state TimeLimitDeal [parallel]
    en,du:
    [TimeDrHeatLevel,TimeoutDrFlag] = TimeoutFunction(HeatAdj_TimeOutPrm,HeatRunMaxTime,ComDrHeatLevel);
    [TimePaHeatLevel,TimeoutPaFlag] = TimeoutFunction1(HeatAdj_TimeOutPrm,HeatRunMaxTime,ComPaHeatLevel);
    [Time3rdHeatLevel,Timeout3rdFlag] = TimeoutFunction2(HeatAdj_TimeOutPrm,HeatRunMaxTime,Com3rdHeatLevel,SwTimeout);
    settings: executionOrder=3
  state [Level,TimeoutFlag] = TimeoutFunction1(TimeoutPrm,MaxTime,InLevel) [function]
  state [Level,TimeoutFlag] = TimeoutFunction2(TimeoutPrm,MaxTime,InLevel,SwTimeout) [function]
  state [StopReason,CANStopReason] = StopFunction(ComStop,Timeout,ComCANStop) [function]
  state StopReasonDeal [parallel]
    en,du:
    [DrHeatStopReason,DrCANHeatStopReason] = StopFunction(ComDrStopReason,TimeoutDrFlag,ComCANDrStopReason);
    [PaHeatStopReason,PaCANHeatStopReason] = StopFunction1(ComPaStopReason,TimeoutPaFlag,ComCANPaStopReason);
    [ThirdHeatStopReason,ThirdCANHeatStopReason] = StopFunction2(Com3rdStopReason,Timeout3rdFlag,ComCANPaStopReason);
    settings: executionOrder=4
  state [StopReason,CANStopReason] = StopFunction1(ComStop,Timeout,ComCANStop) [function]
  state [StopReason,CANStopReason] = StopFunction2(ComStop,Timeout,ComCANStop) [function]
  state [Level,Type] = DiagnoseFunction(DiagCommand,InLevel,CurrentType) [function]
  state DiagnoseCtrlDeal [parallel]
    en,du:
    [DiagDrHeatLevel,HeatDriverRunType] = DiagnoseFunction(HeatAdj_DriverDiagCmd,TimeDrHeatLevel,OrgHeatDriverRunType);
    [DiagPaHeatLevel,HeatPassengerRunType] = DiagnoseFunction1(HeatAdj_PassengerDiagCmd,TimePaHeatLevel, OrgHeatPassengerRunType);
    [Diag3rdHeatLevel,HeatThirdRunType] = DiagnoseFunction2(HeatAdj_ThirdDiagCmd,Time3rdHeatLevel,OrgHeatThirdRunType);
    settings: executionOrder=5
  state [Level,Type] = DiagnoseFunction1(DiagCommand,InLevel,CurrentType) [function]
  state [Level,Type] = DiagnoseFunction2(DiagCommand,InLevel,CurrentType) [function]
  data: MixFlg function_input uint8; Valid function_input uint8; OutValid function_output; OriginalLevel function_input; Error function_input; OppositeCmd function_input; CarType function_input; Level function_output; StopReason function_output; Heat_CanMessageLostFlag function_input; Heat_RecoverDefaultFlag function_input; CANStopReason function_output; OriginalLevel function_input; Error function_input; OppositeCmd function_input; CarType function_input; Level function_output; StopReason function_output; Heat_CanMessageLostFlag function_input; Heat_RecoverDefaultFlag function_input; CANStopReason function_output; OriginalLevel function_input; Error function_input; OppositeCmd function_input; CarType function_input; Level function_output; StopReason function_output; Heat_CanMessageLostFlag function_input; Heat_RecoverDefaultFlag function_input; CANStopReason function_output; TimeoutPrm function_input; MaxTime function_input uint32; InLevel function_input; Level function_output; TimeoutFlag function_output; TimeoutPrm function_input; MaxTime function_input uint32; InLevel function_input; Level function_output; TimeoutFlag function_output; TimeoutPrm function_input; MaxTime function_input uint32; InLevel function_input; Level function_output; TimeoutFlag function_output; SwTimeout function_input uint32; ComStop function_input; Timeout function_input; StopReason function_output; ComCANStop function_input Enum: enHeatStopReason; CANStopReason function_output; ComStop function_input; Timeout function_input; StopReason function_output; ComCANStop function_input Enum: enHeatStopReason; CANStopReason function_output; ComStop function_input; Timeout function_input; StopReason function_output; ComCANStop function_input Enum: enHeatStopReason; CANStopReason function_output; DiagCommand function_input; InLevel function_input; Level function_output; CurrentType function_input; Type function_output; DiagCommand function_input; InLevel function_input; Level function_output; CurrentType function_input; Type function_output; DiagCommand function_input; InLevel function_input; Level function_output; CurrentType function_input; Type function_output; OriginalDrHeatLevel input; OriginalPaHeatLevel input; Original3rdHeatLevel input; HeatAdj_VoltMode input; DriverHeatError input; PassengerHeatError input; ThirdHeatError input; DriverVentilateValid input; PassengerVentilateValid input; ThirdVentilateValid input; HeatAdj_CarType input; HeatAdj_RecoverDefaultFlag input; HeatAdj_HeatMsgLostFlag input; HeatAdj_TimeOutPrm input; HeatRunMaxTime input; ComDrHeatLevel local Enum: enHeatLvlSts; ComPaHeatLevel local Enum: enHeatLvlSts; Com3rdHeatLevel local Enum: enHeatLvlSts; TimeDrHeatLevel local Enum: enHeatLvlSts; TimePaHeatLevel local Enum: enHeatLvlSts; Time3rdHeatLevel local Enum: enHeatLvlSts; ComDrStopReason local Enum: enHeatStopReason; ComPaStopReason local Enum: enHeatStopReason; Com3rdStopReason local Enum: enHeatStopReason; TimeoutDrFlag local uint8; TimeoutPaFlag local uint8; Timeout3rdFlag local uint8; DrHeatStopReason output Enum: enHeatStopReason; ThirdHeatStopReason output Enum: enHeatStopReason; PaHeatStopReason output Enum: enHeatStopReason; DiagDrHeatLevel output Enum: enHeatLvlSts; DiagPaHeatLevel output Enum: enHeatLvlSts; Diag3rdHeatLevel output Enum: enHeatLvlSts; HeatDriverRunType output Enum: enHeatType; HeatPassengerRunType output Enum: enHeatType; HeatThirdRunType output Enum: enHeatType; OrgHeatDriverRunType input; OrgHeatPassengerRunType input; OrgHeatThirdRunType input; HeatAdj_DriverDiagCmd input; HeatAdj_PassengerDiagCmd input; HeatAdj_ThirdDiagCmd input; ComCANDrStopReason local Enum: enHeatStopReason; ComCANPaStopReason local Enum: enHeatStopReason; ComCAN3rdStopReason local Enum: enHeatStopReason; DrCANHeatStopReason output Enum: enHeatStopReason; PaCANHeatStopReason output Enum: enHeatStopReason; ThirdCANHeatStopReason output Enum: enHeatStopReason; Driver_MixConflicFlg input; Passenger_MixConflicFlg input; Third_MixConflicFlg input; LocalDriverVentilateValid local uint8; LocalPassengerVentilateValid local uint8; LocalThirdVentilateValid local uint8; SwTimeout input

== stateflow chart Appl_HeatAdj_CtrlModel/LogicCtrl/LocalAdjustCtrl/HeatLevelDeal ==
  state IVISwCan = CANAquireFunction(HeatLevel,IVISwsHeat,PowerMode) [function]
  state Level = LevelAquireFunction(EnableCfg,CarTypeCfg,CAN_Message,DisableSts,ComPCFlag,CanLvl,Type) [function]
  state Level = LevelAquireFunction3(EnableCfg,CarTypeCfg,CAN_Message,DisableSts,ComPCFlag,CanLvl,Type) [function]
  state Level = SwLevelAquireFunction1(EnableCfg,CAN_Message,DisableSts,ComPCFlag) [function]
  state Level = LevelAquireFunction1(EnableCfg,CarTypeCfg,CAN_Message,DisableSts,ComPCFlag,CanLvl,Type) [function]
  state Level = LevelAquireFunction4(EnableCfg,CarTypeCfg,CAN_Message,DisableSts,ComPCFlag,CanLvl,Type) [function]
  state Level = SwLevelAquireFunction(EnableCfg,CAN_Message,DisableSts,ComPCFlag) [function]
  state Level = LevelAquireFunction2(EnableCfg,CarTypeCfg,CAN_Message,DisableSts,ComPCFlag,CanLvl,Type) [function]
  state Level = LevelAquireFunction5(EnableCfg,CarTypeCfg,CAN_Message,DisableSts,ComPCFlag,CanLvl,Type) [function]
  state DriverHeatLevelDeal [parallel]
    settings: executionOrder=1
    state HMI_HeatFunction [parallel]
      settings: executionOrder=1
      (default) -> (junction 36)
      DriverHeatLevelDeal.HMI_HeatFunction -> (junction 36)
      (junction 36) -> (junction 163)
      (junction 163) -> (junction 39) : {LocalDrHMIHeatLevel = LevelAquireFunction(DrHeatConfig, ...
          | HeatAdj_CarType, DriverHMI_Message,...
          | HeatAdj_DrHeatStopReason,ComPCSatisfiedFlag,HeatAdj_CanDrvHeatLvl,FALSE);}
      (junction 39) -> (junction 41) [order 1] : /* 主驾加热大屏判断 */
          | [LocalDrHMIHeatLevel <= enHeatLvlSts.EN_HEAT_LVL_3]
      (junction 39) -> (junction 45) [order 2]
      (junction 41) -> (junction 43) : {OrgHeatDriverRunType = enHeatType.EN_HEAT_TYPE_HMI;
          | OriginalDrHeatLevel = LocalDrHMIHeatLevel;}
      (junction 43) -> (junction 45)
      (junction 45) -> (junction 172)
    state Tbox_HeatFunction [parallel]
      settings: executionOrder=2
      (default) -> (junction 65)
      DriverHeatLevelDeal.Tbox_HeatFunction -> (junction 65)
      (junction 65) -> (junction 67) [order 1] : [TRUE == RemoteModeFlag]
      (junction 65) -> (junction 176) [order 2] : {LocalDrTboxHeatLevel = 0xFF;}
      (junction 67) -> (junction 62) : {LocalDrTboxHeatLevel = LevelAquireFunction1(DrHeatConfig, ...
          | HeatAdj_CarType,DriverTbox_Message, ...
          | HeatAdj_DrHeatStopReason,ComPCSatisfiedFlag, ...
          | HeatAdj_CanDrvHeatLvl,TRUE);}
      (junction 62) -> (junction 176)
      (junction 176) -> (junction 70)
      (junction 70) -> (junction 56) [order 1] : /* 主驾加热远程判断 */
          | [LocalDrTboxHeatLevel <= enHeatLvlSts.EN_HEAT_LVL_3]
      (junction 70) -> (junction 59) [order 2]
      (junction 56) -> (junction 60) : {OrgHeatDriverRunType = enHeatType.EN_HEAT_TYPE_TBOX;
          | OriginalDrHeatLevel = LocalDrTboxHeatLevel;}
      (junction 60) -> (junction 59)
      (junction 59) -> (junction 183)
  state ThirdHeatLevelDeal [parallel]
    settings: executionOrder=3
    state BM400_ThirdHeatLevelDeal
      state Tbox_HeatFunction [parallel]
        settings: executionOrder=2
        (default) -> (junction 270)
        ThirdHeatLevelDeal.BM400_ThirdHeatLevelDeal.Tbox_HeatFunction -> (junction 270)
        (junction 270) -> (junction 293) [order 1] : [TRUE == RemoteModeFlag]
        (junction 270) -> (junction 295) [order 2] : {Local3rdTboxHeatLevel = 0xFF;}
        (junction 293) -> (junction 312) : {Local3rdTboxHeatLevel = LevelAquireFunction5(ThirdHeatConfig, ...
            | HeatAdj_CarType,ThirdTbox_Message, ...
            | HeatAdj_ThirdHeatStopReason,ComPCSatisfiedFlag ,...
            | HeatAdj_CanThirdHeatLvl,TRUE);}
        (junction 312) -> (junction 295)
        (junction 295) -> (junction 275)
        (junction 275) -> (junction 314) [order 1] : /* 三排加热远程判断 */
            | [Local3rdTboxHeatLevel <= enHeatLvlSts.EN_HEAT_LVL_3]
        (junction 275) -> (junction 304) [order 2]
        (junction 314) -> (junction 302) : {OrgHeatThirdRunType = enHeatType.EN_HEAT_TYPE_TBOX;
            | Original3rdHeatLevel = Local3rdTboxHeatLevel;}
        (junction 302) -> (junction 304)
        (junction 304) -> (junction 257)
      state HMI_HeatFunction [parallel]
        settings: executionOrder=1
        (default) -> (junction 285)
        ThirdHeatLevelDeal.BM400_ThirdHeatLevelDeal.HMI_HeatFunction -> (junction 285)
        (junction 285) -> (junction 254)
        (junction 254) -> (junction 265) : {Local3rdHMIHeatLevel = LevelAquireFunction4(ThirdHeatConfig, ...
            | HeatAdj_CarType,ThirdHMI_Message, ...
            | HeatAdj_ThirdHeatStopReason,ComPCSatisfiedFlag, ...
            | HeatAdj_CanThirdHeatLvl,FALSE);}
        (junction 265) -> (junction 267) [order 1] : /* 三排加热大屏判断 */
            | [Local3rdHMIHeatLevel <= enHeatLvlSts.EN_HEAT_LVL_3]
        (junction 265) -> (junction 255) [order 2]
        (junction 267) -> (junction 264) : {OrgHeatThirdRunType = enHeatType.EN_HEAT_TYPE_HMI;
            | Original3rdHeatLevel = Local3rdHMIHeatLevel;}
        (junction 264) -> (junction 255)
        (junction 255) -> (junction 262)
    state P20_SteerWheeling
      state Tbox_HeatFunction [parallel]
        settings: executionOrder=2
        (default) -> (junction 392)
        ThirdHeatLevelDeal.P20_SteerWheeling.Tbox_HeatFunction -> (junction 392)
        (junction 392) -> (junction 386) [order 1] : [TRUE == RemoteModeFlag]
        (junction 392) -> (junction 378) [order 2] : {Local3rdTboxHeatLevel = 0xFF;}
        (junction 386) -> (junction 387) : {Local3rdTboxHeatLevel = SwLevelAquireFunction1(ThirdHeatConfig, ...
            | ThirdTbox_Message, ...
            | HeatAdj_ThirdHeatStopReason,ComPCSatisfiedFlag);}
        (junction 387) -> (junction 378)
        (junction 378) -> (junction 403)
        (junction 403) -> (junction 397) [order 1] : /* 三排加热远程判断 */
            | [Local3rdTboxHeatLevel <= enHeatLvlSts.EN_HEAT_LVL_3]
        (junction 403) -> (junction 396) [order 2]
        (junction 397) -> (junction 382) : {OrgHeatThirdRunType = enHeatType.EN_HEAT_TYPE_TBOX;
            | Original3rdHeatLevel = Local3rdTboxHeatLevel;}
        (junction 382) -> (junction 396)
        (junction 396) -> (junction 395)
      state HMI_HeatFunction [parallel]
        settings: executionOrder=1
        (default) -> (junction 345)
        ThirdHeatLevelDeal.P20_SteerWheeling.HMI_HeatFunction -> (junction 345)
        (junction 345) -> (junction 348) : {HMI_CanMessage = CANAquireFunction(HeatAdj_D_SimuIndex_ThirdHeat, ...
            | ThirdHMI_Message,HeatAdj_PowerMode);}
        (junction 348) -> (junction 368) : {Local3rdHMIHeatLevel = SwLevelAquireFunction(ThirdHeatConfig,...
            | HMI_CanMessage,...
            | HeatAdj_ThirdHeatStopReason,ComPCSatisfiedFlag);}
        (junction 368) -> (junction 370) [order 1] : /* 三排加热大屏判断 */
            | [Local3rdHMIHeatLevel <= enHeatLvlSts.EN_HEAT_LVL_3]
        (junction 368) -> (junction 369) [order 2]
        (junction 370) -> (junction 367) : {OrgHeatThirdRunType = enHeatType.EN_HEAT_TYPE_HMI;
            | Original3rdHeatLevel = Local3rdHMIHeatLevel;}
        (junction 367) -> (junction 369)
        (junction 369) -> (junction 372)
    (default) -> BM400_ThirdHeatLevelDeal
    BM400_ThirdHeatLevelDeal -> P20_SteerWheeling : /*P20车型方向盘加热*/
        | [enProjectType.EN_PROJECT_P20 == HeatAdj_CarType]
    P20_SteerWheeling -> BM400_ThirdHeatLevelDeal : /*三排加热*/
        | [enProjectType.EN_PROJECT_P20 != HeatAdj_CarType]
  state PassengerHeatLevelDeal [parallel]
    settings: executionOrder=2
    state Tbox_HeatFunction [parallel]
      settings: executionOrder=2
      (default) -> (junction 209)
      PassengerHeatLevelDeal.Tbox_HeatFunction -> (junction 209)
      (junction 209) -> (junction 250) [order 1] : [TRUE == RemoteModeFlag]
      (junction 209) -> (junction 246) [order 2] : {LocalPaTboxHeatLevel = 0xFF;}
      (junction 250) -> (junction 197) : {LocalPaTboxHeatLevel = LevelAquireFunction3(PaHeatConfig, ...
          | HeatAdj_CarType,PassengerTbox_Message, ...
          | HeatAdj_PaHeatStopReason,ComPCSatisfiedFlag, ...
          | HeatAdj_CanPasHeatLvl,TRUE);}
      (junction 197) -> (junction 246)
      (junction 246) -> (junction 206)
      (junction 206) -> (junction 193) [order 1] : /* 副驾加热远程判断 */
          | [LocalPaTboxHeatLevel <= enHeatLvlSts.EN_HEAT_LVL_3]
      (junction 206) -> (junction 194) [order 2]
      (junction 193) -> (junction 195) : {OrgHeatPassengerRunType = enHeatType.EN_HEAT_TYPE_TBOX;
          | OriginalPaHeatLevel = LocalPaTboxHeatLevel;}
      (junction 195) -> (junction 194)
      (junction 194) -> (junction 228)
    state HMI_HeatFunction [parallel]
      settings: executionOrder=1
      (default) -> (junction 251)
      PassengerHeatLevelDeal.HMI_HeatFunction -> (junction 251)
      (junction 251) -> (junction 222)
      (junction 222) -> (junction 221) : {LocalPaHMIHeatLevel = LevelAquireFunction2(PaHeatConfig, ...
          | HeatAdj_CarType,PassengerHMI_Message, ...
          | HeatAdj_PaHeatStopReason,ComPCSatisfiedFlag, ...
          | HeatAdj_CanPasHeatLvl,FALSE);}
      (junction 221) -> (junction 215) [order 1] : /* 副驾加热大屏判断*/
          | [LocalPaHMIHeatLevel <= enHeatLvlSts.EN_HEAT_LVL_3]
      (junction 221) -> (junction 218) [order 2]
      (junction 215) -> (junction 219) : {OrgHeatPassengerRunType = enHeatType.EN_HEAT_TYPE_HMI;
          | OriginalPaHeatLevel = LocalPaHMIHeatLevel;}
      (junction 219) -> (junction 218)
      (junction 218) -> (junction 236)
  data: HeatLevel function_input; IVISwCan function_output; IVISwsHeat function_input; PowerMode function_input; EnableCfg function_input; Level function_output; CarTypeCfg function_input; CAN_Message function_input; DisableSts function_input; ComPCFlag function_input uint8; CanLvl function_input uint8; Type function_input uint8; EnableCfg function_input; Level function_output; CarTypeCfg function_input; CAN_Message function_input; DisableSts function_input; ComPCFlag function_input uint8; CanLvl function_input uint8; Type function_input uint8; EnableCfg function_input; Level function_output; CAN_Message function_input; DisableSts function_input; ComPCFlag function_input uint8; EnableCfg function_input; Level function_output; CarTypeCfg function_input; CAN_Message function_input; DisableSts function_input; ComPCFlag function_input uint8; CanLvl function_input uint8; Type function_input uint8; EnableCfg function_input; Level function_output; CarTypeCfg function_input; CAN_Message function_input; DisableSts function_input; ComPCFlag function_input uint8; CanLvl function_input uint8; Type function_input uint8; EnableCfg function_input; Level function_output; CAN_Message function_input; DisableSts function_input; ComPCFlag function_input uint8; EnableCfg function_input; Level function_output; CarTypeCfg function_input; CAN_Message function_input; DisableSts function_input; ComPCFlag function_input uint8; CanLvl function_input uint8; Type function_input uint8; EnableCfg function_input; Level function_output; CarTypeCfg function_input; CAN_Message function_input; DisableSts function_input; ComPCFlag function_input uint8; CanLvl function_input uint8; Type function_input uint8; DrHeatConfig input; PaHeatConfig input; ThirdHeatConfig input; HeatAdj_DrHeatStopReason input; HeatAdj_PaHeatStopReason input; HeatAdj_ThirdHeatStopReason input; HeatAdj_PowerMode input; HeatAdj_CarType input; DriverHMI_Message input; DriverTbox_Message input; PassengerHMI_Message input; PassengerTbox_Message input; ThirdHMI_Message input; ThirdTbox_Message input; OriginalDrHeatLevel output Enum: enHeatLvlSts; OrgHeatDriverRunType output Enum: enHeatType; RemoteModeFlag input; TRUE parameter; OriginalPaHeatLevel output Enum: enHeatLvlSts; OrgHeatPassengerRunType output Enum: enHeatType; Original3rdHeatLevel output Enum: enHeatLvlSts; OrgHeatThirdRunType output Enum: enHeatType; LocalDrHMIHeatLevel local uint8 =255; HeatAdj_D_SimuIndex_ThirdHeat input; HMI_CanMessage local uint8; Local3rdTboxHeatLevel local uint8 =255; Local3rdHMIHeatLevel local uint8 =255; LocalPaTboxHeatLevel local uint8 =255; LocalPaHMIHeatLevel local uint8 =255; LocalDrTboxHeatLevel local uint8 =255; ComPCSatisfiedFlag input; HeatAdj_CanDrvHeatLvl input; HeatAdj_CanPasHeatLvl input; HeatAdj_CanThirdHeatLvl input; FALSE parameter
